simulink model "Simulink_Clarke_Transfomation_and_Park_Transformation"  (Simulink 10.1)
settings: Solver=VariableStepAuto  StartTime=0.0  StopTime=10.0  RelTol=1e-3
libraries: simulink x1
settings Model: Creator=Wilson_hhx  LastModifiedBy=Wilson_hhx
settings DataIOCC: SaveFormat=Dataset  ReturnWorkspaceOutputs=on
settings OptimizationCC: LifeSpan=auto
settings DebuggingCC: UnderspecifiedInitializationDetection=Simplified  MergeDetectMultiDrivingBlocksExec=error  SFUnexpectedBacktrackingDiag=error  SFNoUnconditionalDefaultTransitionDiag=error  SFExecutionAtInitializationDiag=warning  ArithmeticOperatorsInVariantConditions=error
settings HardwareCC: ProdBitPerPointer=64  ProdBitPerSizeT=64  ProdBitPerPtrDiffT=64  ProdLargestAtomicFloat=Float  ProdIntDivRoundTo=Zero  ProdEndianess=LittleEndian  ProdWordSize=64  ProdHWDeviceType=Intel->x86-64 (Windows64)
settings ModelReferenceCC: PropagateSignalLabelsOutOfModel=on
settings SFSimCC: SimUseLocalCustomCode=on  CustomCodeUndefinedFunction=FilterOut
settings RTWCC: RTWUseLocalCustomCode=on
settings CodeAppCC: StateflowObjectComments=off
settings GRTTargetCC: TargetLangStandard=C99 (ISO)  CombineOutputUpdateFcns=on  GRTInterface=off
settings ConfigComp: CovMetricSettings=dwe  CovHtmlReporting=off  CovSaveCumulativeToWorkspaceVar=off  CovSaveSingleToWorkspaceVar=off  CovExternalEMLEnable=on

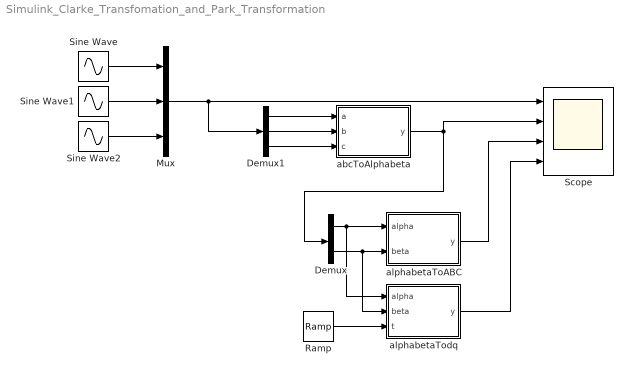
== system Simulink_Clarke_Transfomation_and_Park_Transformation ==
  Demux : Demux  Outputs=2
  Demux1 : Demux  Outputs=3
  Mux : Mux  Inputs=3
  Ramp : simulink/Sources/Ramp  slope=1  start=0  InitialOutput=0
  Scope : Scope  NumInputPorts=4
  Sine Wave : Sin  Frequency=10  Phase=pi/2  SampleTime=0
  Sine Wave1 : Sin  Frequency=10  Phase=pi/2-2*pi/3  SampleTime=0
  Sine Wave2 : Sin  Frequency=10  Phase=pi/2+2*pi/3  SampleTime=0
  abcToAlphabeta : MATLAB Function  TreatAsAtomicUnit=on
  alphabetaToABC : MATLAB Function  TreatAsAtomicUnit=on
  alphabetaTodq : MATLAB Function  TreatAsAtomicUnit=on
  wires:
  Sine Wave2/1 -> Mux/3
  Demux1/3 -> abcToAlphabeta/3(c)
  alphabetaToABC/1(y) -> Scope/3
  Sine Wave1/1 -> Mux/2
  Sine Wave/1 -> Mux/1
  Demux/2 -> alphabetaTodq/2(beta), alphabetaToABC/2(beta)
  Demux1/1 -> abcToAlphabeta/1(a)
  Mux/1 -> Demux1/1, Scope/1
  Demux/1 -> alphabetaTodq/1(alpha), alphabetaToABC/1(alpha)
  Demux1/2 -> abcToAlphabeta/2(b)
  abcToAlphabeta/1(y) -> Demux/1, Scope/2
  Ramp/1 -> alphabetaTodq/3(t)
  alphabetaTodq/1(y) -> Scope/4

== matlab function alphabetaToABC ==
  data: alpha input double; y output double; beta input double
function y = fcn(alpha,beta)

a = alpha;
b = -1/2 * alpha + sqrt(3)/2 * beta;
c = -1/2 * alpha - sqrt(3)/2 * beta;
 
y = [a;b;c];

== matlab function abcToAlphabeta ==
  data: a input double; y output double; b input double; c input double
function y = fcn(a,b,c)

alpha = a - b/2 - c/2;
beta = sqrt(3)/2 * (b - c);
y = (2/3)*[alpha;beta];

== matlab function alphabetaTodq ==
  data: alpha input double; y output double; beta input double; t input double
function y = fcn(alpha,beta,t)

%f = 10;
%T = 1/f;
%w = 2*pi/T
w = 10;
d =  alpha*cos(w*t) + beta*sin(w*t);
q = -alpha*sin(w*t) + beta*cos(w*t);
 
y = [d;q];
